simulink model "Bands8"  (R2018a)
settings: Solver=VariableStepAuto  StartTime=0.0  StopTime=0.007  RelTol=1e-3
undefined symbols (not defined in the file): fdesignblkfcn, G1, G2, G3, G4, G5, G6, G7, G8, gcbh, get, T
libraries: dspsrcs4 x1, dspxfrm3 x1, dspobslib x1
(part 2 of 3)

== system Bands8/Filter Bank /Filter 4/Bandpass Filter ==
  In : Inport
  Generated Filter Block : DiscreteFir  Tag=BlockMethodSubSystem  Coefficients=[-5.30821769158583662e-08 1.39314081737948182e-07 5.41312478502524594e-07 4.86136672338418073e-07 -7.96499196494103078e-07 -2.42334954088225584e-06 -1.5351290337091759e-06 3.2136341825850962e-06 7.35084357515251779e-06 3.05746676520898631e-06 -9.95580910173521477e-06 -1.75780100130185448e-05 -3.6035257523428706e-06 2.54174137595758371e-05 3.51380253464884796e-05 -7.73738553051543951e-07 -5.56291412505974329e-05 -6.01271779548091209e-05 1.75854348213130179e-05 0.000106856070269362508 8.82531531318072666e-05 -5.80190075650452577e-05 -0.000182598412057078714 -0.000108380900863090047 0.000135132077452252585 0.00027922408460884804 0.000101402536827980929 -0.000259482429584985159 -0.000381383619960095797 -4.20140851290521581e-05 0.000432460744600594469 0.000459278437902259622 -9.5460157754566379e-05 -0.000638958482731849086 -0.000470258746629898406 0.000327367360602756055 0.000842356824289018061 0.000366615188313596419 -0.000649295017153990396 -0.000985434251625084577 -0.00010956394906791167 0.00102701242644657586 0.000999969791041195946 -0.000313375309208497634 -0.00139484203588836745 -0.000825273732456746254 0.000873204313229052217 0.00166552186765287456 0.000432061672370809551 -0.00149351076785194693 -0.00175231480915308377 0.00015572060842223209 0.00205965351366623438 0.00159912318804657227 -0.000850523051024917962 -0.00244472666297297723 -0.00120936455823856702 0.00151027710776925031 0.00254750671941166712 0.000661665623882588144 -0.00196958653823885773 -0.0023310753383089999 -0.000102057998397751004 0.00208743342415047307 0.00184717372654995249 -0.000291021688731959679 -0.00179749447299426676 -0.0012330983131586318 0.000362451475533147923 0.00114243273058247199 0.000675872635465359366 -4.01556570738553588e-05 -0.000275473855878565323 -0.000350700761418277617 -0.000623640085072828731 -0.000577916416422045867 0.000353019453583895801 0.00144976026227562355 0.00119066844474382378 -0.000650389036222980368 -0.00217671887145664059 -0.00141468977179822365 0.00107766529035621108 0.00254370001373110553 0.00124071182407995122 -0.00138541721310411563 -0.00238548090734601054 -0.000809914275279410281 0.00133103105806634502 0.00170328497594346537 0.00036547416699127933 -0.000781952802680303664 -0.000679538224777078174 -0.000155804918784333446 -0.000210023541483689231 -0.000377092678330671839 0.000323911606410355059 0.00139918150664343358 0.00114265502982478502 -0.000828772232244089058 -0.00241503326532845888 -0.00140533958374749915 0.00143788040706721164 0.00289277231588474376 0.00115730048765743136 -0.00180493144648723224 -0.00261874465622023711 -0.000607170740888487255 0.00161125283890593287 0.00163156769826277659 9.85012601815445332e-05 -0.000718116800492914881 -0.000230494146999192474 4.09530112864431469e-05 -0.000735766475422064783 -0.00112357544745852653 0.00034010221443167896 0.00234284365759225349 0.00198408281883988681 -0.00111769885099965321 -0.00355329492017253694 -0.00210386810484999983 0.00190952854665029617 0.0038811268958521359 0.00154902638510606466 -0.0022165844741849957 -0.00311097405183421256 -0.000683282473995757041 0.0016431663330456574 0.00141599537538057447 1.5675070636809239e-05 -0.000106627351300604987 0.000675083460044442144 3.46605355457298977e-05 -0.00205994122775666815 -0.00246483173420189309 0.000641776975986285973 0.00417452797013677553 0.00336314043514932296 -0.00174473861102722471 -0.00543771630610335576 -0.00314036499658772346 0.00264691057500181888 0.00524985176908511313 0.00204266384805466307 -0.00264733348956602138 -0.00348609398256280066 -0.00070313589679186128 0.00130351459560600199 0.000603640374650680502 -0.00013313863965918685 0.00129885709150754031 0.0024861399410328641 -3.47694585790582364e-05 -0.00447151762764871636 -0.00475213837712714932 0.00118143311261999879 0.00710825532122491728 0.00546109563607505028 -0.00268812114995703238 -0.00808512459402259062 -0.00450350125929041816 0.00355282912908186236 0.00673085630309314641 0.00247325221109657859 -0.00282102461747457635 -0.00317140669306542437 ...(+6612 chars)]  InputProcessing=Columns as channels (frame based)
  Out : Outport
  wires:
  In/1 -> Generated Filter Block/1
  Generated Filter Block/1 -> Out/1

== system Bands8/Filter Bank /Filter 5/Bandpass Filter ==
  In : Inport
  Generated Filter Block : DiscreteFir  Tag=BlockMethodSubSystem  Coefficients=[-3.46206934279781941e-08 1.04584736309709578e-07 2.86000138223426292e-07 -1.86360452750481946e-07 -1.00479819912692813e-06 -4.58378020198468485e-08 2.49926543315572681e-06 1.36886011603291473e-06 -4.80471223575628475e-06 -5.10946052532882561e-06 7.19550963629337726e-06 1.29767954749277572e-05 -7.56143829976706144e-06 -2.64157195795122925e-05 1.92983294803127946e-06 4.54048419785621425e-05 1.54610974671495855e-05 -6.68563523222181377e-05 -5.11043338341316003e-05 8.31025552410708044e-05 0.00010993024254111115 -8.12523016202484178e-05 -0.000191953003084082845 4.42978934728459469e-05 0.000288625522298755334 4.54034190036943765e-05 -0.000380242784362144987 -0.000200327237421322601 0.000436001289550690704 0.000420701608869883273 -0.000418029061519345762 -0.00068819702323382121 0.000289727215296948278 0.0009630290421639156 -2.7246871500187669e-05 -0.00118688276841606905 -0.000368709643552797041 0.00129279824098340874 0.000864697178433025183 -0.00122100429463348073 -0.00139386468352808556 0.000937233154772074378 0.00186523652367555012 -0.000448166856959109528 -0.00218251550775325079 -0.00019173934446715745 0.00226855382405479009 0.000886196601913511665 -0.00208878813363693426 -0.00151641467172833094 0.00166589865267965324 0.00196996127478176429 -0.00107952476223769126 -0.00217131067683506724 0.000448985417675493094 0.00210441033758928522 9.74738357844225528e-05 -0.00181898987728397942 -0.000458223288607253337 0.00141697433785756884 0.000587185604236794439 -0.00102197876198883552 -0.000505923290284493953 0.000741195799991749109 0.000293749235632528567 -0.000632550969778400874 -5.83438332917382782e-05 0.000689047252762856901 -0.000103206726746712262 -0.000846586216486119912 0.000138748671239108493 0.00101294722529970765 -5.74935183915716935e-05 -0.00110716913717989925 -7.84228984815332216e-05 0.00109376374115315186 0.000184542250535737633 -0.000997355614889683774 -0.000194751317959334134 0.00089061689566397235 9.48060441467483771e-05 -0.000859307406452637949 6.67301620529098211e-05 0.000958555461573901103 -0.000196956052265186404 -0.00117970494595144018 0.000200845987915567337 0.00144428419508538697 -3.02080252199123125e-05 -0.00163122573507523769 -0.00028268055919035591 0.00162907354906602787 0.000624637714495869848 -0.0013924422967358152 -0.00083948345866725828 0.000977214631621166081 0.000792721687508539602 -0.00053498791598942223 -0.000437653065890009356 0.0002628448764537758 -0.000146766701376731701 -0.000323982203013797616 0.00076773840743567549 0.000769992133073395995 -0.00118260479755669351 -0.00149935629552731126 0.00119487616135966184 0.00227578759293931097 -0.000745246585594879418 -0.00280728595689863506 -4.24801160025329916e-05 0.00286055005309831124 0.0008866453348464439 -0.00236667957252073092 -0.00144313456559715873 0.00147199165033073086 0.0014397018755810116 -0.000505262751593662119 -0.000797416211173010078 -0.000135322284305120356 -0.000313527713120960905 0.000137766102740408028 0.00151494887165719945 0.000585831757632825057 -0.00235279697900214572 -0.00183877747755291539 0.00247524855431352497 0.00319053192984980732 -0.00178745996147545777 -0.00412947006039250056 0.000515999322956514888 0.00426461090408113575 0.00085314040291926724 -0.00349726030056752213 -0.00174973183804534365 0.00208815661912012266 0.00174575057557639808 -0.000582174097548321065 -0.000743629198557197043 -0.000391346962409602685 -0.000955588158835048683 0.000370794848758403215 0.0027434019609695365 0.000733434887128816952 -0.00393035612862495647 -0.00257197375754057017 0.00402505155328493867 0.00446655376368643511 -0.00295357070071784614 -0.00566602865864113559 0.00112255273137480075 0.00565331933677036286 0.000713402610925520484 -0.00437883414555715646 -0.0017403750007757453 0.00231643607325650444 0.00142122750595131487 -0.000304122103854635598 0.000258355674637044351 -0.00078081330782616093 -0.00274473853352199095 0.000388467967130704276 0.0051072211448565958 0.00144655496241283136 -0.00640321674250788481 -0.00407508140107300243 ...(+7005 chars)]  InputProcessing=Columns as channels (frame based)
  Out : Outport
  wires:
  In/1 -> Generated Filter Block/1
  Generated Filter Block/1 -> Out/1

== system Bands8/Filter Bank /Filter 6/Bandpass Filter ==
  In : Inport
  Generated Filter Block : DiscreteFir  Tag=BlockMethodSubSystem  Coefficients=[-4.10860504220904449e-08 -6.27470342553619745e-08 2.03477482842761722e-07 1.46995749521951169e-07 -6.87671523728120039e-07 -1.20305926169604678e-07 1.7859584204428882e-06 -4.6289985851228649e-07 -3.76184059033069542e-06 2.52258310308734223e-06 6.54810014667471715e-06 -7.53655210477210937e-06 -9.23609828862783109e-06 1.73447277310125988e-05 9.45204511352574906e-06 -3.34924673894719169e-05 -2.86146530520322383e-06 5.60163982426290665e-05 -1.6807033032872431e-05 -8.17924677241105058e-05 5.67763784102097357e-05 0.00010288049349580812 -0.000122966418138351351 -0.000105618777369700381 0.000216536159313563672 7.1391273854728548e-05 -0.000329868350954240258 2.01590260947978462e-05 0.000443271402755562156 -0.000185271035576450161 -0.000524097159250950487 0.000428327239149358351 0.000529899870163720067 -0.000734130789669923249 -0.000416487396564405553 0.00106298247717574517 0.000150249859113151934 -0.00135151897139388082 0.000277695279108953997 0.00152137514767000789 -0.000839637892584915117 -0.00149570216114324134 0.00146648177783577707 0.00122079670691204291 -0.0020539689731466867 -0.000687397674256142745 0.00248129160726114116 -5.53555127549162796e-05 -0.00263959619696811252 0.000899794380852076857 0.00246381168824316666 -0.00169692187632478975 -0.00195841932089054968 0.00228941991081460213 0.00120760809638816892 -0.00255324257983461896 -0.000363439199497392687 0.0024361409731272262 -0.000388219146616462438 -0.00198021933291638464 0.00087674221072042203 0.00131869625388801267 -0.000997187667605676977 -0.000644171399155612123 0.000745856608306689995 0.000155019763486513297 -0.00022737766429444057 4.98852535066955543e-06 -0.000372344635491658033 0.00020561996451914764 0.000841837935974267177 -0.000708473518897807038 -0.00101224318795397629 0.00132681879574479645 0.00081555532196883379 -0.00184196740294163158 -0.000311693346033850485 0.00206773289616090077 -0.000327708095033296676 -0.00191769873967497146 0.000876281552880490869 0.00144045626677070026 -0.00113296052385130817 -0.000807586140009724195 0.000997242362822593981 0.000255487910084893014 -0.000511310365087918836 3.66582622710960254e-07 -0.000149135332375898154 0.000151796838636442241 0.000735364455414109271 -0.000672089775134336988 -0.00101770335571265292 0.00137666178137427209 0.000875724886272477424 -0.00200186340902161518 -0.000351221963919855803 0.00230359557471921045 -0.00035939856762561527 -0.00215507292012611209 0.000974449533493306776 0.00160408598715739434 -0.00123467826570015666 -0.000864093783002594967 0.00100889395160145895 0.000238114429706682418 -0.000354839916023780126 -1.41566164241096708e-06 -0.000492464129009005484 0.000287658510068706445 0.00120531547181116001 -0.00102510261068467835 -0.0014915505329267352 0.0019525417046410789 0.00121701842930175327 -0.00271418672756393916 -0.000471554098173668744 0.00300017512150802055 -0.000452869546902859809 -0.00267802620868981111 0.00116922071890306046 0.00185994526930811487 -0.00134961523758317229 -0.000873287620871859935 0.000866057241496989553 0.000139264238761769877 0.000141917458050814539 -3.60284823255680186e-06 -0.00130641367500902109 0.000586305550707772209 0.00216883264276765235 -0.00171483373160428716 -0.0023657982541430817 0.0029750637196946858 0.0017890090512031095 -0.00386758922229661194 -0.000649853522728177408 0.00401170461558310494 -0.00058569986261994343 -0.00331484679631194063 0.00137449072815455805 0.0020334077531869079 -0.00131969187117368636 -0.000690847970777161316 0.000349679683299966343 -0.00012338991099310301 0.00122681400982352015 -1.54524060503518285e-06 -0.00282226570156581934 0.00110992484463539091 0.00379795329001244393 -0.00283208406401724237 -0.00373111723978420068 0.00450887136463909346 0.00261159854382472063 -0.00544878267977462818 -0.000878960891145944391 0.00521930063024696016 -0.000728406910983486256 -0.00385155504352600962 0.00146328012153526966 0.00186443618959016314 -0.00088680434726425071 -8.32734431540487494e-05 -0.000919585717824818465 -0.000686680578970007087 ...(+7281 chars)]  InputProcessing=Columns as channels (frame based)
  Out : Outport
  wires:
  In/1 -> Generated Filter Block/1
  Generated Filter Block/1 -> Out/1

== system Bands8/Filter Bank /Filter 7/Bandpass Filter ==
  In : Inport
  Generated Filter Block : DiscreteFir  Tag=BlockMethodSubSystem  Coefficients=[3.55219413124343128e-08 -3.99522153998837631e-08 -5.74334936233819283e-08 2.03665249498638788e-07 -1.4401234024952182e-07 -2.78646038711110786e-07 6.89176430447719753e-07 -3.35964944845543691e-07 -9.09040175627137098e-07 1.78619380402060039e-06 -6.22332035672071951e-07 -2.31130290158061403e-06 3.89767756152112028e-06 -1.02310939105229017e-06 -4.93064935751708912e-06 7.58765330215307115e-06 -1.74068548916333537e-06 -9.19156402832104134e-06 1.37466818888495846e-05 -3.47530472387566084e-06 -1.54564301330071192e-05 2.40168974551570799e-05 -7.87012931747852341e-06 -2.42040570545393435e-05 4.15178351925066754e-05 -1.78677589958755389e-05 -3.66677347017263841e-05 7.17854726031380254e-05 -3.76282366489089103e-05 -5.60509395165036852e-05 0.000123542872764120283 -7.15619259652003234e-05 -8.91851428584613555e-05 0.000208664110387668739 -0.00012219283225812621 -0.000148048056233350241 0.000340562876946949339 -0.000186996016724657585 -0.00025013201749682953 0.000530477968551402285 -0.000255047419905198014 -0.000416451276712017857 0.000781808792002837709 -0.000305024566185482056 -0.000666310540084823688 0.00108372138315217682 -0.000306451427159901537 -0.00100895347667928235 0.00140634211769084393 -0.000225676840603394576 -0.00143375791892207897 0.00170045445895424256 -3.67134006218124836e-05 -0.0019022494149990494 0.00190414305876215363 0.000265085624129419127 -0.00234611818619662963 0.00195700039971309029 0.000650799896732689271 -0.00267486956958491208 0.00181956392717372165 0.00105281529153237606 -0.00279432242762227973 0.00149248251713582402 0.00137186785365466359 -0.00263321913397745414 0.00102788627845777397 0.00149829032507886118 -0.00217091173292349856 0.000525912317145648192 0.00134442163996073192 -0.00145623000014980528 0.000113013265297926338 0.000879566853938703198 -0.00060798149583255693 -9.4994669281187646e-05 0.000155108053203474903 0.000208027257492139351 -3.51308106235132716e-05 -0.000692408827466997959 0.000822697446207928517 0.000270236011506735973 -0.00146704047559209193 0.00111644599459296287 0.000705514799995940337 -0.00196527812079063096 0.00106314341290603977 0.00108739349693567759 -0.00204024754297842982 0.000746775608613033754 0.00122103173371058147 -0.0016567108977005088 0.000339534169618676586 0.000971282543719830731 -0.00091455122370111394 4.34011196782498271e-05 0.00032393285730457984 -2.67047544721841709e-05 1.25576681832466428e-05 -0.000588948482292576698 0.000746776728992729457 0.000284953044618992861 -0.00151574513067167529 0.00118890520492542675 0.000752513846087451196 -0.0021619739573840507 0.00120762337181511224 0.00118833660213161531 -0.00229403977892586337 0.000875377456832487954 0.0013282926595803927 -0.00183249985118626928 0.000405139373777963331 0.000981072971713275099 -0.000896003337267271436 6.54134397358430131e-05 0.000124533239891651867 0.000227969534752477121 6.31120813047289422e-05 -0.00105447612556198197 0.00118209623973595124 0.000440998767236368576 -0.00220196033854468641 0.00167465641945380682 0.00103652088202556996 -0.00291429080747410141 0.00159852418522718693 0.0015285077397958226 -0.00289218529323701911 0.00108141739205588764 0.00156327025893312154 -0.00207104287746981593 0.000438618710338464042 0.000915396768478881078 -0.00066980232926372495 3.86221565495452156e-05 -0.000383131588476090003 0.000871744607416939047 0.000131916799050745426 -0.00200726553334992612 0.00205274305251248838 0.000715776186496652322 -0.00342583829562781352 0.00250988933698005276 0.00150103719521899612 -0.00409038862995757084 0.00217294537799166913 0.00200951185418661755 -0.0036576291799988777 0.00130490081696882712 0.00177552106939919577 -0.00215376253423928913 0.0003974734976272445 0.000574431103913125422 -2.79570992200322589e-06 -4.61201059602883668e-05 -0.0014216730639115974 0.00210890648745145357 0.000245217858057432229 -0.00364204622062439757 0.00349108386516006845 0.00114909956312295039 -0.00529224823386062471 0.00373161222099370297 0.00215528723953379003 -0.00565360302809551039 0.00288112468923756556 ...(+7706 chars)]  InputProcessing=Columns as channels (frame based)
  Out : Outport
  wires:
  In/1 -> Generated Filter Block/1
  Generated Filter Block/1 -> Out/1
